simulink model "OmniSimulinkModel"  (R2020b)
settings: Solver=FixedStepAuto  StartTime=0.0  StopTime=5  FixedStep=0.001  RelTol=1e-3
libraries: simulink_extras x3
settings Model: Creator=USER  LastModifiedBy=김예온

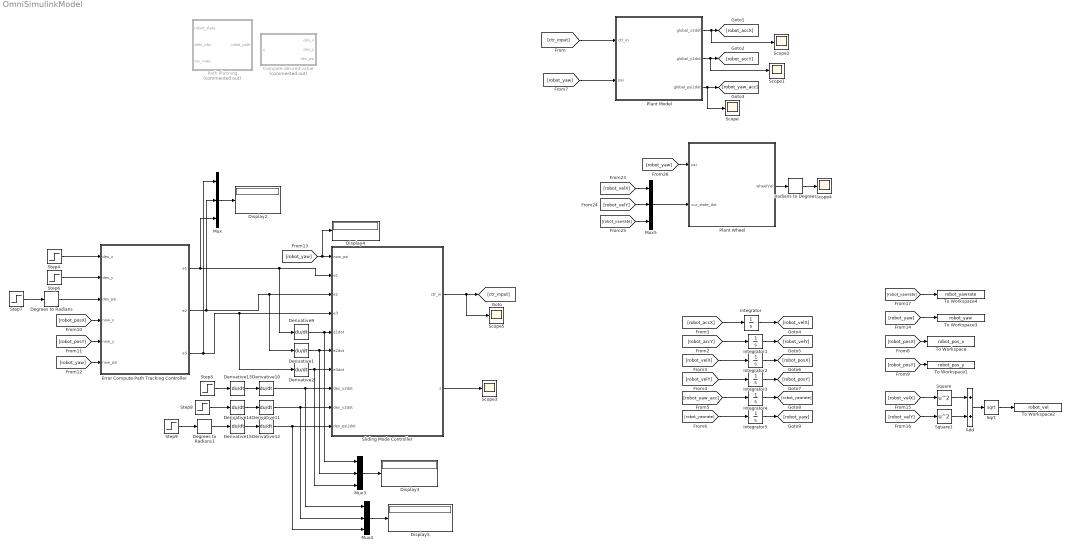
== system OmniSimulinkModel ==
  Add : Sum
  Compute desired value : MATLAB Function  Commented=on  TreatAsAtomicUnit=on
  Degrees to Radians : simulink_extras/Transformations/Degrees to Radians
  Degrees to Radians1 : simulink_extras/Transformations/Degrees to Radians
  Derivative{1..2,9..15} (9 alike) : Derivative
  Display{2..5} (4 alike) : Display
  Error Compute Path Tracking Controller : MATLAB Function  TreatAsAtomicUnit=on
  Integrator{,1..5} (6 alike) : Integrator
  Mux{,3..5} (4 alike) : Mux  Inputs=3
  Path Planning : MATLAB Function  Commented=on  TreatAsAtomicUnit=on
  Plant Model : MATLAB Function  TreatAsAtomicUnit=on
  Plant Wheel : MATLAB Function  TreatAsAtomicUnit=on
  Radians to Degrees : simulink_extras/Transformations/Radians to Degrees
  Scope{,1..5} (6 alike) : Scope
  Sliding Mode Controller : MATLAB Function  TreatAsAtomicUnit=on
  Sqrt : Sqrt  SaturateOnIntegerOverflow=on
  Square : Math  Operator=square  SaturateOnIntegerOverflow=on
  Square1 : Math  Operator=square  SaturateOnIntegerOverflow=on
  Step4 : Step  Time=0  After=3  SampleTime=0
  Step5 : Step  Time=0  After=3  SampleTime=0
  Step{6..9} (4 alike) : Step  Time=0  After=0  SampleTime=0
  To Workspace : ToWorkspace  VariableName=robot_pos_x  SaveFormat=Timeseries  SampleTime=-1
  To Workspace1 : ToWorkspace  VariableName=robot_pos_y  SaveFormat=Timeseries  SampleTime=-1
  To Workspace2 : ToWorkspace  VariableName=robot_vel  SaveFormat=Timeseries  SampleTime=-1
  To Workspace3 : ToWorkspace  VariableName=robot_yaw  SaveFormat=Timeseries  SampleTime=-1
  To Workspace4 : ToWorkspace  VariableName=robot_yawrate  SaveFormat=Timeseries  SampleTime=-1
  wires:
  [ctr_input] -> Plant Model/1(ctr_in)
  Plant Model/1(global_x2dot) -> Scope2/1, [robot_accX]
  Plant Model/2(global_y2dot) -> Scope1/1, [robot_accY]
  Plant Model/3(global_psi2dot) -> Scope/1, [robot_yaw_acc]
  Integrator/1 -> [robot_velX]
  Integrator1/1 -> [robot_velY]
  Integrator2/1 -> [robot_posX]
  Integrator3/1 -> [robot_posY]
  Integrator4/1 -> [robot_yawrate]
  Integrator5/1 -> [robot_yaw]
  [robot_yaw] -> Plant Model/2(psi)
  [robot_posX] -> To Workspace/1
  [robot_posY] -> To Workspace1/1
  [robot_posX] -> Error Compute Path Tracking Controller/4(now_x)
  [robot_posY] -> Error Compute Path Tracking Controller/5(now_y)
  [robot_yaw] -> Error Compute Path Tracking Controller/6(now_psi)
  Add/1 -> Sqrt/1
  Square/1 -> Add/1
  Square1/1 -> Add/2
  [robot_velX] -> Square/1
  [robot_velY] -> Square1/1
  Sqrt/1 -> To Workspace2/1
  Sliding Mode Controller/1(ctr_in) -> Scope5/1, [ctr_input]
  [robot_yaw] -> Display4/1, Sliding Mode Controller/1(now_psi)
  Error Compute Path Tracking Controller/2(e2) -> Mux/2, Sliding Mode Controller/3(e2), Derivative1/1
  Error Compute Path Tracking Controller/3(e3) -> Mux/1, Sliding Mode Controller/4(e3), Derivative2/1
  Step4/1 -> Error Compute Path Tracking Controller/1(des_x)
  Step6/1 -> Error Compute Path Tracking Controller/2(des_y)
  Degrees to Radians/1 -> Error Compute Path Tracking Controller/3(des_psi)
  Derivative15/1 -> Derivative12/1
  Derivative13/1 -> Derivative10/1
  Derivative14/1 -> Derivative11/1
  Derivative12/1 -> Mux4/3, Sliding Mode Controller/10(des_psi2dot)
  Derivative10/1 -> Mux4/1, Sliding Mode Controller/8(des_x2dot)
  Derivative9/1 -> Mux3/1, Sliding Mode Controller/5(e1dot)
  Derivative1/1 -> Mux3/2, Sliding Mode Controller/6(e2dot)
  Derivative2/1 -> Mux3/3, Sliding Mode Controller/7(e3dot)
  [robot_accX] -> Integrator/1
  [robot_accY] -> Integrator1/1
  [robot_velX] -> Integrator2/1
  [robot_velY] -> Integrator3/1
  [robot_yaw_acc] -> Integrator4/1
  [robot_yawrate] -> Integrator5/1
  Mux/1 -> Display2/1
  Error Compute Path Tracking Controller/1(e1) -> Mux/3, Sliding Mode Controller/2(e1), Derivative9/1
  Step5/1 -> Derivative13/1
  [robot_yaw] -> To Workspace3/1
  [robot_yawrate] -> To Workspace4/1
  Sliding Mode Controller/2(s) -> Scope3/1
  Degrees to Radians1/1 -> Derivative15/1
  Step8/1 -> Derivative14/1
  Mux3/1 -> Display3/1
  Mux4/1 -> Display5/1
  Derivative11/1 -> Mux4/2, Sliding Mode Controller/9(des_y2dot)
  Step9/1 -> Degrees to Radians1/1
  Step7/1 -> Degrees to Radians/1
  [robot_yawrate] -> Mux5/3
  [robot_velY] -> Mux5/2
  [robot_velX] -> Mux5/1
  Mux5/1 -> Plant Wheel/2(cur_state_dot)
  [robot_yaw] -> Plant Wheel/1(psi)
  Radians to Degrees/1 -> Scope4/1
  Plant Wheel/1(wheelVel) -> Radians to Degrees/1

== matlab function OmniSimulinkModel/Plant Model ==
  data: ctr_in input; global_x2dot output; psi input; global_y2dot output; global_psi2dot output
function [global_x2dot, global_y2dot, global_psi2dot]= fcn(ctr_in, psi)
R = 0.05;   % wheel radius [m]
J1 = 0.095;%0.000625;  % nominal inertial of wheel [kgm^2]
H = [0 J1/2 0 J1/2;
     -J1/2 0 -J1/2 0;
     0 J1/2 0 J1/2;
     -J1/2 0 -J1/2 0];
hpsi_mat = h_psi(psi);
% global position Q = [x y psi]^T
% global state = Q2dot
% wheelspeed = [theta1dot theta2dot theta3dot theta4dot]^T
% global_state = R/(4*J1) * hpsi_mat * (H*ctr_in + J1*wheelacc);
global_state = R/(4*J1) * hpsi_mat * ctr_in;
% 
% if(isnan(global_state(1)))
%     global_state(1) = 0;
% end
% 
% if(isnan(global_state(2)))
%     global_state(2) = 0;
% end
%     
% if(isnan(global_state(3)))
%     global_state(3) = 0;
% end

global_x2dot = global_state(1);
global_y2dot = global_state(2);
global_psi2dot = global_state(3);
end

function mat = h_psi(psi)
% returns psi 3x4 matrix
psi = psi + pi/4;
root2 = sqrt(2);

% third row should be 1/(a+b) which will be 1/(2*rou)
mat = [-root2*sin(psi) root2*cos(psi) -root2*sin(psi) root2*cos(psi);
        root2*cos(psi) root2*sin(psi) root2*cos(psi) root2*sin(psi);
        10/3 -10/3 -10/3 10/3];
end

== matlab function OmniSimulinkModel/Compute desired value ==
  data: u input; des_x output; des_y output; des_psi output
function [des_x, des_y, des_psi]= fcn(u)

des_x=0;
des_y=0; 
des_psi=0;

== matlab function OmniSimulinkModel/Error Compute Path Tracking Controller ==
  data: des_x input; e1 output; des_y input; des_psi input; now_x input; now_y input; now_psi input; e2 output; e3 output
function [e1, e2, e3]= fcn(des_x, des_y, des_psi, now_x, now_y, now_psi)
e1 = -(now_x - des_x);
e2 = -(now_y - des_y);
e3 = -(now_psi - des_psi);
end

== matlab function OmniSimulinkModel/Path Planning ==
  data: robot_state input; ideal_path output; detc_obs input; rec_map input
function ideal_path = fcn(robot_state, detc_obs, rec_map)

ideal_path = robot_state;

== matlab function OmniSimulinkModel/Sliding Mode Controller ==
  data: now_psi input; ctr_in output; e1 input; e2 input; e3 input; e1dot input; e2dot input; e3dot input; des_x2dot input; des_y2dot input; des_psi2dot input; s output
function [ctr_in, s]= fcn(now_psi, e1, e2, e3, e1dot, e2dot, e3dot, des_x2dot, des_y2dot, des_psi2dot)
J1 = 0.095;%0.000625;  % nominal inertial of wheel [kgm^2]
R = 0.05;   % wheel radius [m]
p = 5;
q = 3;
lamda1 = 1.25;%1.5;
lamda2 = 1.25;%1.5;
lamda3 = 1.25;%1.5;
errdot = [e1dot; e2dot; e3dot];
Qr2dot = [des_x2dot; des_y2dot; des_psi2dot];
e1dot = abs(e1dot);
e2dot = abs(e2dot);
e3dot = abs(e3dot);
% sliding mode
s = [e1 + lamda1*(e1dot)^(p/q); e2 + lamda2*(e2dot)^(p/q); e3 + lamda3*(e3dot)^(p/q);];

% if(isinf(e1dot))
%     e1dot = 0;
% end
% if(isinf(e2dot))
%     e2dot = 0;
% end
% if(isinf(e3dot))
%     e3dot = 0;
% end
% if(isinf(des_x2dot))
%     des_x2dot = 0;
% end
% if(isinf(des_y2dot))
%     des_y2dot = 0;
% end
% if(isinf(des_psi2dot))
%     des_psi2dot = 0;
% end

% important!!
M_inv = [0 0 0;
        0 0 0;
        0 0 0];
if(e1dot ~= 0)
    M_inv(1,1) = q/(p*lamda1)*e1dot^(1-(p/q));
end
if(e2dot ~= 0)
    M_inv(2,2) = q/(p*lamda2)*e2dot^(1-(p/q));
end
if(e3dot ~= 0)
    M_inv(3,3) = q/(p*lamda3)*e3dot^(1-(p/q));
end


d = 0.5;%25; %[Nm] 
B = [8*d 0 0; 0 8*d 0; 0 0 4*d/0.3];
hpsi_inv_mat = hpsi_inv(now_psi);     
u_eq = 4*J1/R * hpsi_inv_mat * (Qr2dot- M_inv*errdot);
u_r = -hpsi_inv_mat * B * sign(s);

% final control input
ctr_in = u_eq + u_r;

% if(isnan(ctr_temp(1)))
%     ctr_temp(1) = 0;
% end
% if(isnan(ctr_temp(2)))
%     ctr_temp(2) = 0;
% end
% if(isnan(ctr_temp(3)))
%     ctr_temp(3) = 0;
% end
% if(isnan(ctr_temp(4)))
%     ctr_temp(4) = 0;
% end
% ctr_in = ctr_temp;
end

function mat = hpsi_inv(psi)
psi = psi + pi/4;
sqrt2 = sqrt(2);
mat = 0.25 * [-sqrt2*sin(psi) sqrt2*cos(psi) 0.3;
                sqrt2*cos(psi) sqrt2*sin(psi) -0.3;
                -sqrt2*sin(psi) sqrt2*cos(psi) -0.3;
                sqrt2*cos(psi) sqrt2*sin(psi) 0.3];
end

== matlab function OmniSimulinkModel/Plant Wheel ==
  data: psi input; cur_state_dot input; wheelVel output
function wheelVel= fcn(psi, cur_state_dot)
R = 0.05;   % wheel radius [m]
hpsi_inv_mat = hpsi_inv(psi);

wheelVel = 4/R* hpsi_inv_mat * cur_state_dot;
end

function mat = hpsi_inv(psi)
psi = psi + pi/4;
sqrt2 = sqrt(2);
mat = 0.25 * [-sqrt2*sin(psi) sqrt2*cos(psi) 0.3;
                sqrt2*cos(psi) sqrt2*sin(psi) -0.3;
                -sqrt2*sin(psi) sqrt2*cos(psi) -0.3;
                sqrt2*cos(psi) sqrt2*sin(psi) 0.3];
end
